simulink model "exogenous_system"  (R2021b)
settings: Solver=FixedStepAuto  StartTime=0.0  StopTime=30  FixedStep=0.05  RelTol=1e-3
settings Model: Creator=den  LastModifiedBy=den

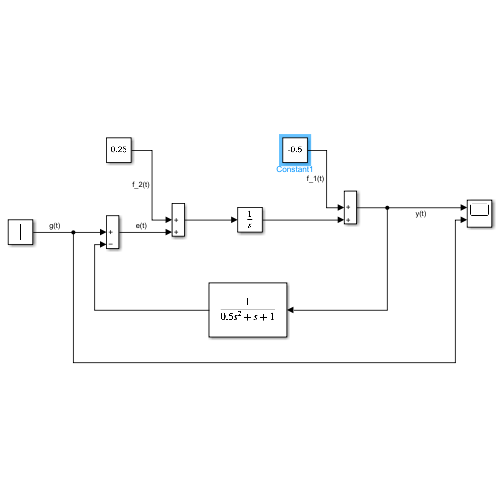
[thumbnail: Simulink's stored preview of the top-level diagram]
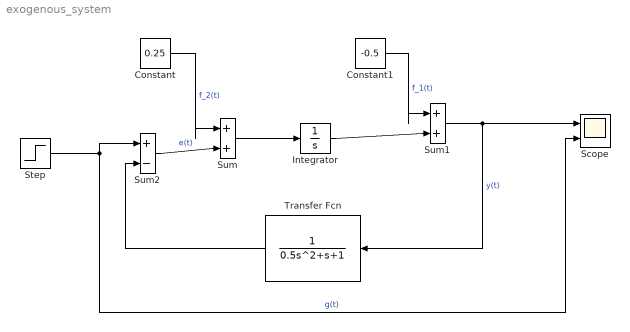
== system exogenous_system ==
  Constant : Constant  Value=0.25
  Constant1 : Constant  Value=-0.5
  Integrator : Integrator
  Scope : Scope  NumInputPorts=2
  Step : Step  Time=0  SampleTime=0
  Sum : Sum  Inputs=|++
  Sum1 : Sum  Inputs=|++
  Sum2 : Sum  Inputs=|+-
  Transfer Fcn : TransferFcn  Denominator=[0.5 1 1]
  wires:
  Integrator/1 -> Sum1/2
  Constant1/1 -> Sum1/1  "f_1(t)"
  Constant/1 -> Sum/1  "f_2(t)"
  Sum/1 -> Integrator/1
  Sum2/1 -> Sum/2  "e(t)"
  Step/1 -> Sum2/1, Scope/2  "g(t)"
  Sum1/1 -> Transfer Fcn/1, Scope/1  "y(t)"
  Transfer Fcn/1 -> Sum2/2
